simulink model "shifter_pulseshaping"  (R2020b)
settings: Solver=VariableStepAuto  StartTime=0.0  StopTime=600e-6  RelTol=1e-3
values from neighbouring files (symbols this model uses):
  a_fir_coeff = [     a_filter_slope_pos  .* ones(1,a_filter_slope_length),                           zeros(1,a_filter_gap_length),      a_filter_slope_neg  .* ones(1,a_filter_slope_length)   ]    [file_pulse_shaping_params.m]    (also in pulse_shaping_params.m)
  hpf_diff_constant = 140e-9    (= 1.4e-07)    [file_pulse_shaping_params.m]    (also in pulse_shaping_params.m = 5e-05)
  lp_coeff = ones(1,ma_length)./ma_length    [file_pulse_shaping_params.m]    (also in pulse_shaping_params.m)
  nakhostin_10_10_k = 2    [file_pulse_shaping_params.m]    (also in pulse_shaping_params.m = 4)
  nakhostin_10_10_l = 64    [file_pulse_shaping_params.m]    (also in pulse_shaping_params.m = 8)
  nakhostin_10_10_M = 1/( exp(sampling_rate/nakhostin_10_10_tau) - 1 )    [file_pulse_shaping_params.m]    (also in pulse_shaping_params.m = 1/( exp(sampling_rate/hpf_diff_constant) - 1 ))
  nakhostin_10_1_eneg = exp(-sampling_rate/2/hpf_diff_constant)    [file_pulse_shaping_params.m]    (also in pulse_shaping_params.m)
  nakhostin_10_1_epos = exp(sampling_rate/2/hpf_diff_constant)    [file_pulse_shaping_params.m]    (also in pulse_shaping_params.m)
  nakhostin_10_1_L = 30    [file_pulse_shaping_params.m]    (also in pulse_shaping_params.m = 16)
  nakhostin_10_3_fir_coeff = [0,ones(1,nakhostin_10_3_L-1)]    [file_pulse_shaping_params.m]    (also in pulse_shaping_params.m)
  nakhostin_10_3_gain = sampling_rate/2/hpf_diff_constant    (= 0.00357142857143)    [file_pulse_shaping_params.m]    (also in pulse_shaping_params.m = 0.001)
  nakhostin_10_3_L = 48    [file_pulse_shaping_params.m]    (also in pulse_shaping_params.m = 8)
  pulse_gen_noise_clock = 50e-9    (= 5e-08)    [file_pulse_shaping_params.m]    (also in pulse_shaping_params.m = 2e-05)
  pulse_gen_period = 1*1e-8    (= 1e-08)    [file_pulse_shaping_params.m]    (also in pulse_shaping_params.m = 0.0001)
  sampling_rate = 1e-9    (= 1e-09)    [file_pulse_shaping_params.m]    (also in pulse_shaping_params.m = 1e-07)
  smooth_derivative_2_coeff = [ones(1,smooth_derivative_2_len), -ones(1,smooth_derivative_2_len)]    [file_pulse_shaping_params.m]    (also in pulse_shaping_params.m)
  smooth_derivative_coeff = [ones(1,smooth_derivative_len), -ones(1,smooth_derivative_len)]    [file_pulse_shaping_params.m]    (also in pulse_shaping_params.m)
libraries: simulink x4, dspstat3 x3
settings Model: Creator=Dickbutt  LastModifiedBy=Dickbutt

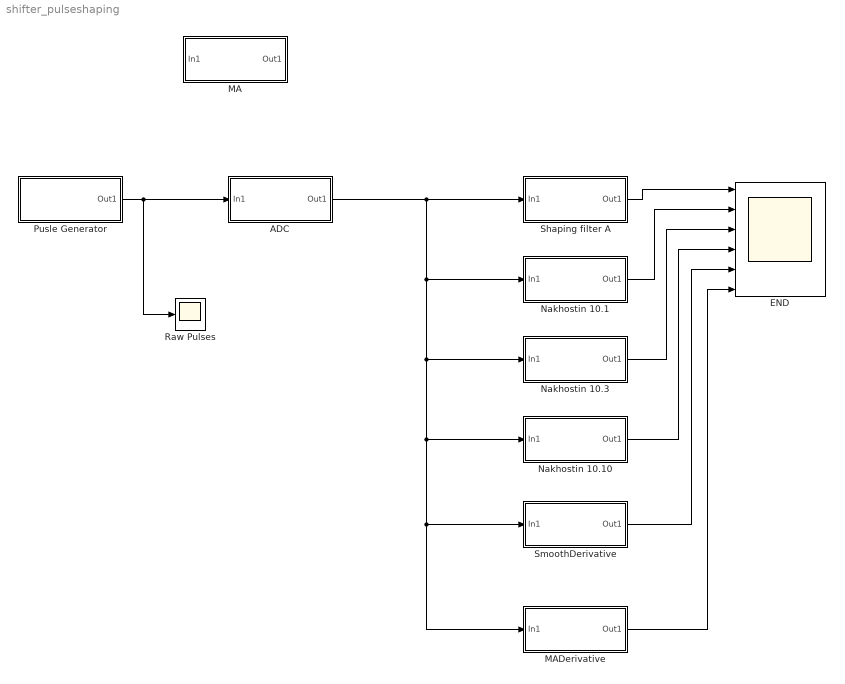
== system shifter_pulseshaping ==
  ADC : Subsystem
  END : Scope  NumInputPorts=6
  MA : Subsystem
  MADerivative : Subsystem
  Nakhostin 10.1 : Subsystem
  Nakhostin 10.10 : Subsystem
  Nakhostin 10.3 : Subsystem
  Pusle Generator : Subsystem
  Raw Pulses : Scope
  Shaping filter A : Subsystem
  SmoothDerivative : Subsystem
  wires:
  Nakhostin 10.1/1(Out1) -> END/2
  Shaping filter A/1(Out1) -> END/1
  Nakhostin 10.3/1(Out1) -> END/3
  Pusle Generator/1(Out1) -> ADC/1(In1), Raw Pulses/1
  ADC/1(Out1) -> MADerivative/1(In1), SmoothDerivative/1(In1), Nakhostin 10.10/1(In1), Nakhostin 10.3/1(In1), Nakhostin 10.1/1(In1), Shaping filter A/1(In1)
  Nakhostin 10.10/1(Out1) -> END/4
  SmoothDerivative/1(Out1) -> END/5
  MADerivative/1(Out1) -> END/6

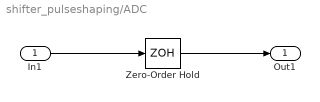
== system shifter_pulseshaping/ADC ==
  In1 : Inport
  Zero-Order Hold : ZeroOrderHold  SampleTime=sampling_rate
  Out1 : Outport
  wires:
  In1/1 -> Zero-Order Hold/1
  Zero-Order Hold/1 -> Out1/1

== system shifter_pulseshaping/MA ==
  In1 : Inport
  Discrete FIR Filter : DiscreteFir  Coefficients=lp_coeff
  Out1 : Outport
  wires:
  In1/1 -> Discrete FIR Filter/1
  Discrete FIR Filter/1 -> Out1/1

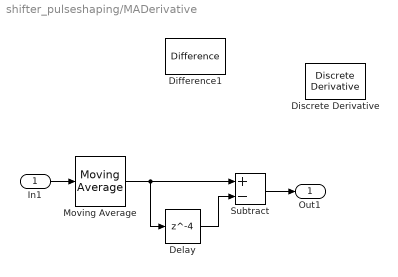
== system shifter_pulseshaping/MADerivative ==
  In1 : Inport
  Delay : Delay  DelayLength=4  InitialCondition=0
  Difference1 : simulink/Discrete/Difference  ICPrevInput=0.0  OutMin=[]  OutMax=[]  OutDataType=fixdt(1, 16)  OutScaling=2^-10  DoSatur=off
  Discrete Derivative : simulink/Discrete/Discrete Derivative  gainval=1.0  ICPrevScaledInput=0.0  OutMin=[]  OutMax=[]  OutDataType=fixdt(1, 16)  OutScaling=2^-10  DoSatur=off
  Moving Average : dspstat3/Moving Average  Method=Sliding window  ForgettingFactorPort=off  SpecifyWindowLength=on  WindowLength=8  ForgettingFactor=0.9  SimulateUsing=Code generation
  Subtract : Sum  Inputs=+-
  Out1 : Outport
  wires:
  In1/1 -> Moving Average/1
  Subtract/1 -> Out1/1
  Moving Average/1 -> Delay/1, Subtract/1
  Delay/1 -> Subtract/2

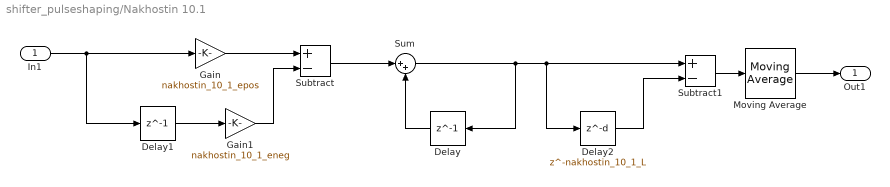
== system shifter_pulseshaping/Nakhostin 10.1 ==
  In1 : Inport
  Delay : Delay  DelayLength=1  InitialCondition=0
  Delay1 : Delay  DelayLength=1  InitialCondition=0
  Delay2 : Delay  DelayLength=nakhostin_10_1_L  InitialCondition=0
  Gain : Gain  Gain=nakhostin_10_1_epos
  Gain1 : Gain  Gain=nakhostin_10_1_eneg
  Moving Average : dspstat3/Moving Average  Method=Sliding window  ForgettingFactorPort=off  SpecifyWindowLength=on  WindowLength=nakhostin_10_1_MA_order  ForgettingFactor=0.9  SimulateUsing=Code generation
  Subtract : Sum  Inputs=+-
  Subtract1 : Sum  Inputs=+-
  Sum : Sum  Inputs=|++
  Out1 : Outport
  wires:
  Delay1/1 -> Gain1/1
  Gain1/1 -> Subtract/2
  Gain/1 -> Subtract/1
  Delay/1 -> Sum/2
  In1/1 -> Delay1/1, Gain/1
  Subtract/1 -> Sum/1
  Sum/1 -> Delay2/1, Subtract1/1, Delay/1
  Delay2/1 -> Subtract1/2
  Subtract1/1 -> Moving Average/1
  Moving Average/1 -> Out1/1

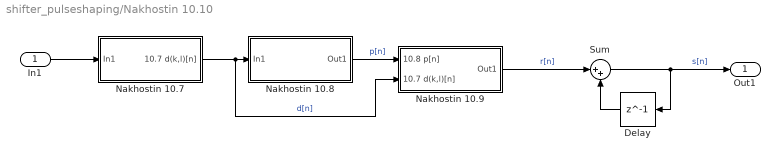
== system shifter_pulseshaping/Nakhostin 10.10 ==
  In1 : Inport
  Delay : Delay  DelayLength=1  InitialCondition=0
  Nakhostin 10.7 : Subsystem
  Nakhostin 10.8 : Subsystem
  Nakhostin 10.9 : Subsystem
  Sum : Sum  Inputs=|++
  Out1 : Outport
  wires:
  In1/1 -> Nakhostin 10.7/1(In1)
  Nakhostin 10.7/1(10.7 d(k,l)[n]) -> Nakhostin 10.9/2(10.7 d(k,l)[n]), Nakhostin 10.8/1(In1)  "d[n]"
  Nakhostin 10.8/1(Out1) -> Nakhostin 10.9/1(10.8 p[n])  "p[n]"
  Nakhostin 10.9/1(Out1) -> Sum/1  "r[n]"
  Sum/1 -> Out1/1, Delay/1  "s[n]"
  Delay/1 -> Sum/2

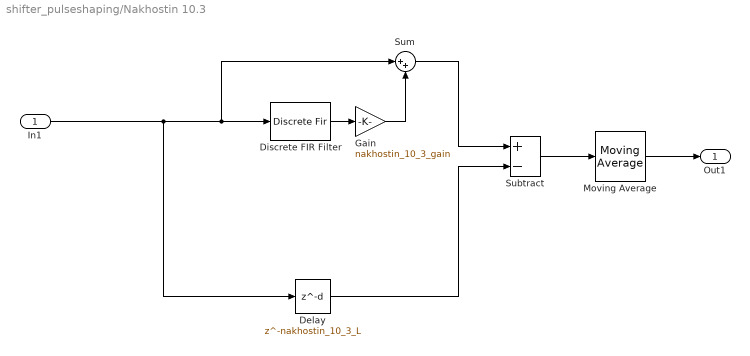
== system shifter_pulseshaping/Nakhostin 10.3 ==
  In1 : Inport
  Delay : Delay  DelayLength=nakhostin_10_3_L  InitialCondition=0
  Discrete FIR Filter : DiscreteFir  Coefficients=nakhostin_10_3_fir_coeff
  Gain : Gain  Gain=nakhostin_10_3_gain
  Moving Average : dspstat3/Moving Average  Method=Sliding window  ForgettingFactorPort=off  SpecifyWindowLength=on  WindowLength=nakhostin_10_3_N  ForgettingFactor=0.9  SimulateUsing=Code generation
  Subtract : Sum  Inputs=+-
  Sum : Sum  Inputs=|++
  Out1 : Outport
  wires:
  In1/1 -> Delay/1, Discrete FIR Filter/1, Sum/1
  Discrete FIR Filter/1 -> Gain/1
  Gain/1 -> Sum/2
  Sum/1 -> Subtract/1
  Delay/1 -> Subtract/2
  Subtract/1 -> Moving Average/1
  Moving Average/1 -> Out1/1

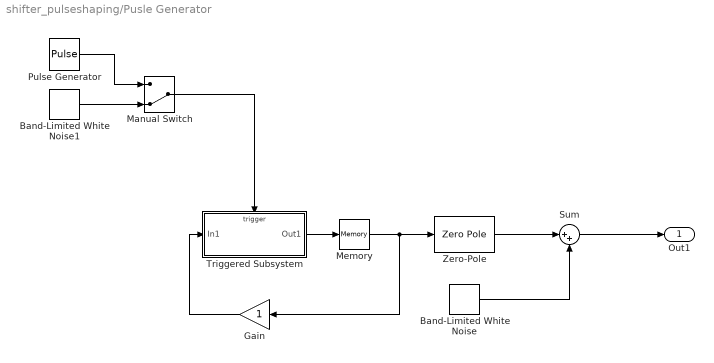
== system shifter_pulseshaping/Pusle Generator ==
  Band-Limited White Noise : simulink/Sources/Band-Limited White Noise  Cov=noise_power  Ts=sampling_rate  seed=[23341]
  Band-Limited White Noise1 : simulink/Sources/Band-Limited White Noise  Cov=[0.5]  Ts=pulse_gen_noise_clock  seed=[23341]
  Gain : Gain
  Manual Switch : ManualSwitch  CurrentSetting=0
  Memory : Memory
  Pulse Generator : DiscretePulseGenerator  PulseType=Time based  Period=pulse_gen_period  PulseWidth=5
  Sum : Sum  Inputs=|++
  Triggered Subsystem : Subsystem  TreatAsAtomicUnit=on
  Zero-Pole : ZeroPole  Zeros=[0]  Poles=[-1/hpf_diff_constant]  Gain=[0.8]
  Out1 : Outport
  wires:
  Pulse Generator/1 -> Manual Switch/1
  Triggered Subsystem/1(Out1) -> Memory/1
  Memory/1 -> Zero-Pole/1, Gain/1
  Gain/1 -> Triggered Subsystem/1(In1)
  Zero-Pole/1 -> Sum/1
  Band-Limited White Noise/1 -> Sum/2
  Sum/1 -> Out1/1
  Band-Limited White Noise1/1 -> Manual Switch/2
  Manual Switch/1 -> Triggered Subsystem/Trigger

== system shifter_pulseshaping/Shaping filter A ==
  In1 : Inport
  Discrete FIR Filter : DiscreteFir  Coefficients=a_fir_coeff
  Out1 : Outport
  wires:
  In1/1 -> Discrete FIR Filter/1
  Discrete FIR Filter/1 -> Out1/1

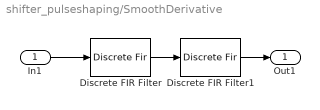
== system shifter_pulseshaping/SmoothDerivative ==
  In1 : Inport
  Discrete FIR Filter : DiscreteFir  Coefficients=smooth_derivative_coeff
  Discrete FIR Filter1 : DiscreteFir  Coefficients=smooth_derivative_2_coeff
  Out1 : Outport
  wires:
  In1/1 -> Discrete FIR Filter/1
  Discrete FIR Filter/1 -> Discrete FIR Filter1/1
  Discrete FIR Filter1/1 -> Out1/1

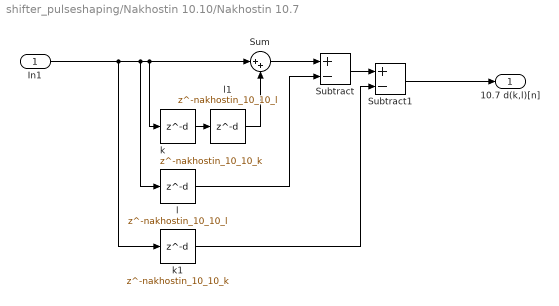
== system shifter_pulseshaping/Nakhostin 10.10/Nakhostin 10.7 ==
  In1 : Inport
  Subtract : Sum  Inputs=+-
  Subtract1 : Sum  Inputs=+-
  Sum : Sum  Inputs=|++
  k : Delay  DelayLength=nakhostin_10_10_k  InitialCondition=0
  k1 : Delay  DelayLength=nakhostin_10_10_k  InitialCondition=0
  l : Delay  DelayLength=nakhostin_10_10_l  InitialCondition=0
  l1 : Delay  DelayLength=nakhostin_10_10_l  InitialCondition=0
  10.7 d(k,l)[n] : Outport
  wires:
  In1/1 -> k1/1, l/1, Sum/1, k/1
  Sum/1 -> Subtract/1
  l/1 -> Subtract/2
  k/1 -> l1/1
  l1/1 -> Sum/2
  k1/1 -> Subtract1/2
  Subtract/1 -> Subtract1/1
  Subtract1/1 -> 10.7 d(k,l)[n]/1

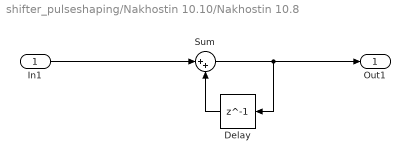
== system shifter_pulseshaping/Nakhostin 10.10/Nakhostin 10.8 ==
  In1 : Inport
  Delay : Delay  DelayLength=1  InitialCondition=0
  Sum : Sum  Inputs=|++
  Out1 : Outport
  wires:
  In1/1 -> Sum/1
  Sum/1 -> Delay/1, Out1/1
  Delay/1 -> Sum/2

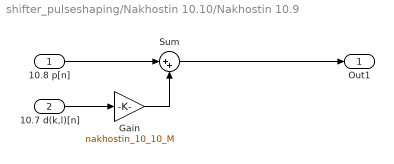
== system shifter_pulseshaping/Nakhostin 10.10/Nakhostin 10.9 ==
  10.8 p[n] : Inport
  10.7 d(k,l)[n] : Inport  Port=2
  Gain : Gain  Gain=nakhostin_10_10_M
  Sum : Sum  Inputs=|++
  Out1 : Outport
  wires:
  10.7 d(k,l)[n]/1 -> Gain/1
  10.8 p[n]/1 -> Sum/1
  Sum/1 -> Out1/1
  Gain/1 -> Sum/2

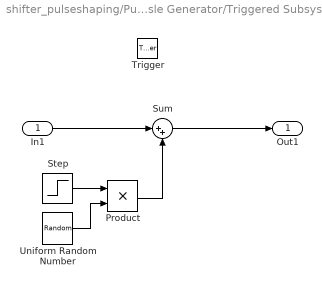
== system shifter_pulseshaping/Pusle Generator/Triggered Subsystem ==
  In1 : Inport
  Trigger : TriggerPort  VariantControl=Variant
  Product : Product
  Step : Step  Time=0
  Sum : Sum  Inputs=|++
  Uniform Random Number : UniformRandomNumber  Minimum=0.1  Maximum=2  Seed=rand(1)
  Out1 : Outport
  wires:
  In1/1 -> Sum/1
  Sum/1 -> Out1/1
  Step/1 -> Product/1
  Uniform Random Number/1 -> Product/2
  Product/1 -> Sum/2
